simulink model "Referenced_battery_pack"  (R2025b)
settings: Solver=ode15s  StartTime=0  StopTime=169.89  MaxStep=1e-2  RelTol=1e-3  AbsTol=1e-6
PreLoadFcn:
  | vehicleData
libraries: batteryecm_lib x280, fl_lib x5, nesl_utility x4, BatteryEstimators x1
(part 1 of 21)
settings Model: PacingRate=0.002200  Creator=muizz  LastModifiedBy=muizz
settings SolverCC: AutoScaleAbsTol=off  MaxConsecutiveMinStep=10000  ZeroCrossAlgorithm=Adaptive
settings DataIOCC: SaveOutput=off  SaveTime=off
settings DebuggingCC: AlgebraicLoopMsg=none  IgnoredZcDiagnostic=none

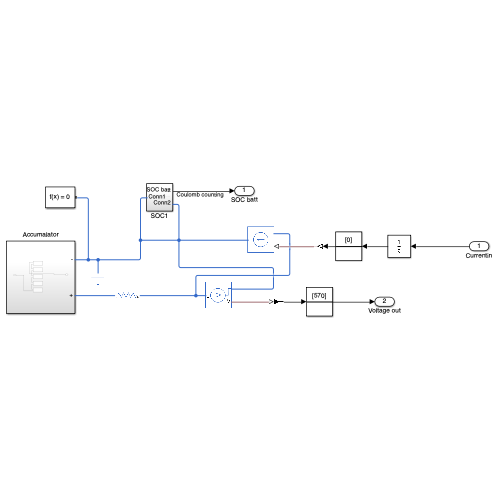
[thumbnail: Simulink's stored preview of the top-level diagram]
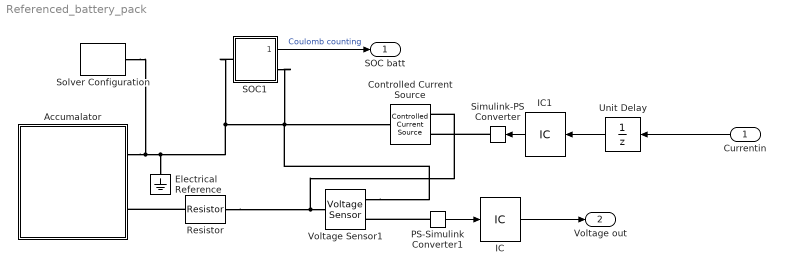
== system Referenced_battery_pack ==
  Currentin : Inport  OutDataTypeStr=double  PortDimensions=1  SampleTime=0.01
  Accumalator : Subsystem
  Controlled Current Source : fl_lib/Electrical/Electrical Sources/Controlled Current Source
  Electrical Reference : fl_lib/Electrical/Electrical Elements/Electrical Reference
  IC : InitialCondition  Value=570
  IC1 : InitialCondition  Value=0
  PS-Simulink Converter1 : nesl_utility/PS-Simulink Converter  PhysicalDomain=network_engine_domain  SubClassName=ps_output  LeftPortType=input  RightPortType=output  PseudoPeriodic=off  Frequencies=[]  VectorFormat=inherit  Unit=inherit  AffineConversion=off
  Resistor : fl_lib/Electrical/Electrical Elements/Resistor  R=1 mOhm  i_specify=off  i_priority=None  i=0 A  i_nominal_specify=off  i_nominal_value=1  i_nominal_unit=A  v_specify=off  v_priority=None  v=0 V  v_nominal_specify=off  v_nominal_value=1  v_nominal_unit=V
  SOC1 : Subsystem
  Simulink-PS Converter : nesl_utility/Simulink-PS Converter  PhysicalDomain=network_engine_domain  SubClassName=ps_input  LeftPortType=input  RightPortType=output  PseudoPeriodic=off  Frequencies=[]  NoiseDistribution=none  NoiseParameters=[]  Unit=A  AffineConversion=off  FilteringAndDerivatives=provide  SimscapeFilterOrder=1  InputFilterTimeConstant=0.001  UdotUserProvided=0
  Solver Configuration : nesl_utility/Solver Configuration  PhysicalDomain=network_engine_domain  SubClassName=solver  LeftPortType=input  RightPortType=generic  Tones=[]  Harmonics=[]  SimulateNoise=off  Profile=off  UseLocalSampling=off  EnableSwitchedLinearOptims=on  FrequencyDomain=off  UseCCode=off  RelTol=0.001  AbsTol=0.001  MinStep=1e-09  ToWorkspace=off  RevertToSquareIcSolve=off  NumHomotopyIterations=100  PhasorMode=off  PhasorModeNumHarmonics=1  ConsistencySolver=NEWTON_XTOL_AFTER_FTOL  IndexReductionMethod=DerivativeReplacement  DoDC=off  ResidualTolerance=1e-09  ConsistencyTolSource=GLOBAL  ConsistencyAbsTol=0.001  ConsistencyRelTol=0.001  ConsistencyTolFactor=0.001  UseLocalSolver=on  LocalSolverChoice=NE_BACKWARD_EULER_ADVANCER  ResolveIndetEquations=on  FunctionEvalNumThread=4  LocalSolverSampleTime=1e-2  DoFixedCost=on  MaxNonlinIter=20  MaxModeIter=2  ComputeImpulses=off  ImpulseIterations=2  LinearAlgebra=auto  LinearAlgebraNumThread=0  EquationFormulation=NE_TIME_EF  DelaysMemoryBudget=1024  AutomaticFiltering=on  FilteringTimeConstant=0.001  PartitionStorageMethod=AS_NEEDED  PartitionMemoryBudget=1024  PartitionMethod=ROBUST  MultibodyUseLocalSolver=off  MultibodyLocalSolverChoice=ODE1  MultibodyLocalSolverSampleTime=0.001
  Unit Delay : UnitDelay  SampleTime=1e-2  HasFrameUpgradeWarning=on
  Voltage Sensor1 : fl_lib/Electrical/Electrical Sensors/Voltage Sensor
  SOC batt : Outport  OutDataTypeStr=double  PortDimensions=1  SampleTime=0.01
  Voltage out : Outport  Port=2  OutDataTypeStr=double  PortDimensions=1  SampleTime=0.01
  wires:
  PS-Simulink Converter1/1 -> IC/1
  SOC1/1(SOC batt) -> SOC batt/1  "Coulomb counting"
  Unit Delay/1 -> IC1/1
  Currentin/1 -> Unit Delay/1
  IC1/1 -> Simulink-PS Converter/1
  IC/1 -> Voltage out/1
  connections:
  Solver Configuration/RConn1 -- Controlled Current Source/LConn1 -- Voltage Sensor1/RConn2 -- SOC1/RConn1 -- SOC1/LConn1 -- Electrical Reference/LConn1 -- Accumalator/LConn1
  Controlled Current Source/RConn2 -- Resistor/LConn1 -- Voltage Sensor1/LConn1
  PS-Simulink Converter1/LConn1 -- Voltage Sensor1/RConn1
  Simulink-PS Converter/RConn1 -- Controlled Current Source/RConn1
  Resistor/RConn1 -- Accumalator/LConn2

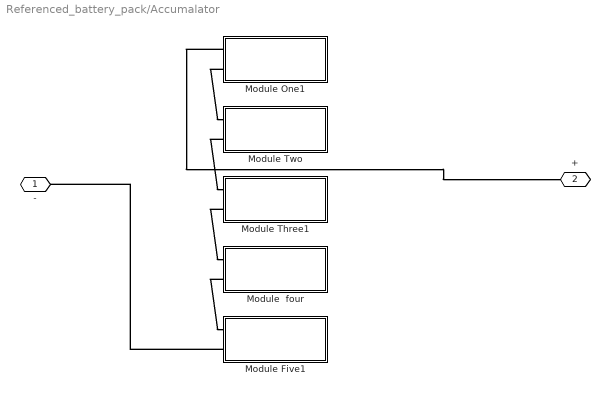
== system Referenced_battery_pack/Accumalator ==
  Module  four : Subsystem
  Module Five1 : Subsystem
  Module One1 : Subsystem
  Module Three1 : Subsystem
  "Module Two " : Subsystem
  - : PMIOPort  Side=Left
  + : PMIOPort  Port=2  Side=Left
  connections:
  "Module Two "/LConn2 -- Module Three1/LConn1
  Module Three1/LConn2 -- Module  four/LConn1
  Module One1/LConn2 -- "Module Two "/LConn1
  Module  four/LConn2 -- Module Five1/LConn1
  Module Five1/LConn2 -- -/RConn1
  Module One1/LConn1 -- +/RConn1

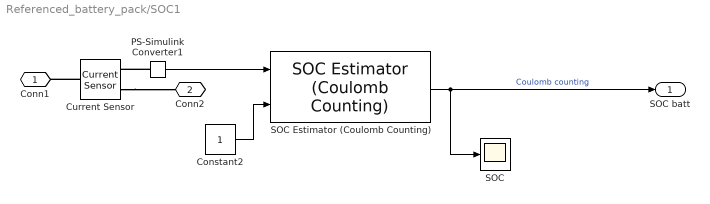
== system Referenced_battery_pack/SOC1 ==
  Constant2 : Constant
  Current Sensor : fl_lib/Electrical/Electrical Sensors/Current Sensor
  PS-Simulink Converter1 : nesl_utility/PS-Simulink Converter  PhysicalDomain=network_engine_domain  SubClassName=ps_output  LeftPortType=input  RightPortType=output  PseudoPeriodic=off  Frequencies=[]  VectorFormat=inherit  Unit=A  AffineConversion=off
  SOC : Scope
      settings: ActiveDisplayYMinimum=-1  ActiveDisplayYMaximum=1  DataLoggingVariableName=ScopeData12
  SOC Estimator (Coulomb Counting) : BatteryEstimators/SOC Estimator (Coulomb Counting)  CurrentInputPartition=on  AH=27  Ts=0.01  DataType=Inherit: auto
      settings: LibrarySourceBlock=|
      | batt_sl_lib/Estimators/SOC Estimator
      | (Coulomb Counting)
  Conn1 : PMIOPort  Side=Left
  Conn2 : PMIOPort  Port=2  Side=Right
  SOC batt : Outport
  wires:
  SOC Estimator (Coulomb Counting)/1 -> SOC batt/1, SOC/1  "Coulomb counting"
  Constant2/1 -> SOC Estimator (Coulomb Counting)/2
  PS-Simulink Converter1/1 -> SOC Estimator (Coulomb Counting)/1
  connections:
  PS-Simulink Converter1/LConn1 -- Current Sensor/RConn1
  Current Sensor/RConn2 -- Conn2/RConn1
  Current Sensor/LConn1 -- Conn1/RConn1
